simulink model "gm_sampleModel1881_sub"  (R2023a)
settings: Solver=VariableStepAuto  StartTime=0.0  StopTime=10.0  RelTol=1e-3
libraries: simulink x2
settings Model: Creator=user1  LastModifiedBy=user1
settings OptimizationCC: BlockReduction=off  ConditionallyExecuteInputs=off
settings DebuggingCC: InheritedTsInSrcMsg=none

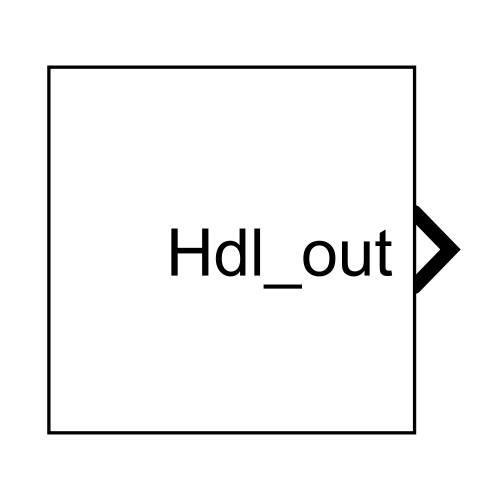
[thumbnail: Simulink's stored preview of the top-level diagram]
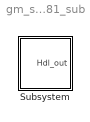
== system gm_sampleModel1881_sub ==
  Subsystem : Subsystem

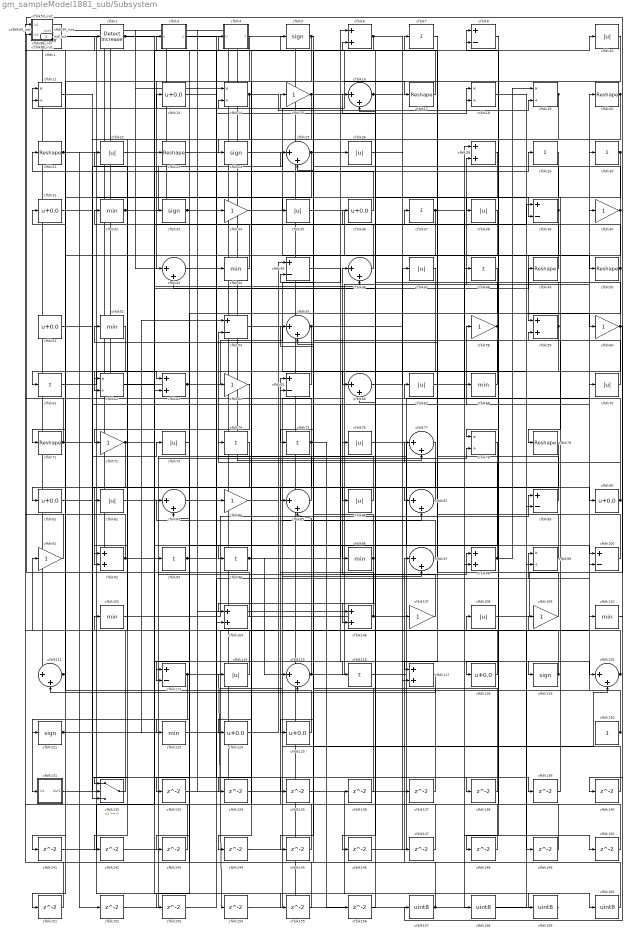
== system gm_sampleModel1881_sub/Subsystem ==
  cfblk1 : simulink/Logic and Bit Operations/Bit Clear  iBit=0
      settings: LibrarySourceBlock=|
      | hdlsllib/Logic and Bit
      | Operations/Bit Clear
  cfblk{10,22,26,35,38,47,67,70,73,76,82,86,108,114} (14 alike) : Abs  OutDataTypeStr=uint8  SaturateOnIntegerOverflow=off
  cfblk{8,39,45,54,65,89,100,113} (8 alike) : Sum  Inputs=+-  OutDataTypeStr=uint8
  cfblk101_inst : Subsystem
  cfblk{32,44,52,68,96,102,110,123} (8 alike) : MinMax  OutDataTypeStr=uint8
  cfblk{6,28,59,63,92,98,104,106,117} (9 alike) : Sum  OutDataTypeStr=uint8
  cfblk105_inst : Subsystem
  cfblk{15,34,40,58,60,64,72,84,91,107,109} (11 alike) : Gain  OutDataTypeStr=uint8
  cfblk{11,14,18..19,62,78,99} (7 alike) : Product  Inputs=*/  OutDataTypeStr=uint8  RndMeth=Zero  SaturateOnIntegerOverflow=on
  cfblk{16,25,43,46,55,66,77,83,85,87,97,111,115,120} (14 alike) : Sum  Inputs=|++  OutDataTypeStr=uint8
  cfblk112_inst : Subsystem
  cfblk{7,29..30,37,48,61,74..75,93..94,116} (11 alike) : Sum  Inputs=+  OutDataTypeStr=uint8
  cfblk{13,31,36,51,81,90,118,124..125} (9 alike) : Bias  Bias=0.0  SaturateOnIntegerOverflow=off
  cfblk{5,24,33,119,121} (5 alike) : Signum
  cfblk130 : Constant  OutDataTypeStr=uint8  SampleTime=-1
  cfblk131 : Subsystem
  cfblk132 : Switch  OutDataTypeStr=uint8  SaturateOnIntegerOverflow=off  InputSameDT=off
  cfblk{133..156} (24 alike) : Delay  SampleTime=1
  cfblk{157..160} (4 alike) : DataTypeConversion  OutDataTypeStr=uint8  SaturateOnIntegerOverflow=off  RndMeth=Floor
  cfblk{17,20..21,23,49..50,71,79} (8 alike) : Reshape
  cfblk2 : simulink/Logic and Bit Operations/Detect Increase  vinit=0.0  OutDataTypeStr=uint8
      settings: LibrarySourceBlock=|
      | hdlsllib/Logic and Bit
      | Operations/Detect
      | Increase
  cfblk3 : Subsystem  mask(Compare To Zero){relop=<=, OutDataTypeStr=uint8, ZeroCross=on}
      mask prompts: relop "Simulink:masks:Operator_MP"; OutDataTypeStr "Simulink:masks:OutputDataType_MP"; ZeroCross "Simulink:masks:EnableZerocrossingDetection_MP"
      mask help: Simulink:masks:CompareToZero_MD
      mask init:
      | OutDataTypeStr = 'uint8';
      | ZeroCross = 'on';
      | blkName = 'sampleModel1881_sub/Subsystem/cfblk3';
      | relop = '<=';
      | setValue = 'fixdt(0, 8)';
      mask TypeOptions relop: == | ~= | < | <= | >= | >
      mask TypeOptions OutDataTypeStr: Simulink:masks:uint8 | Simulink:masks:boolean
      mask Callback ZeroCross: sl('zeroCrossEnable', gcbh);
      mask Display: disp([relop,' 0'])
  cfblk4 : Subsystem  mask(Detect Rise Positive){vinit=double(0), InputProcessing=Elements as channels (sample based), OutDataTypeStr=uint8}
      mask prompts: vinit "Simulink:masks:InitialCondition_MP"; InputProcessing "Simulink:masks:InputProcessing_MP"; OutDataTypeStr "Simulink:masks:OutputDataType_MP"
      mask help: Simulink:masks:DetectRisePositive_MD
      mask init:
      | InputProcessing = 'Elements as channels (sample based)';
      | OutDataTypeStr = 'uint8';
      | vinit = double(0);
      mask TypeOptions InputProcessing: Simulink:masks:ColumnsAsChannelsFrameBased | Simulink:masks:ElementsAsChannelsSampleBased
      mask TypeOptions OutDataTypeStr: Simulink:masks:uint8 | Simulink:masks:boolean
      mask Display: fprintf('U > 0\n&  NOT\nU/z > 0')
  cfblk42_inst : Subsystem
  cfblk53_inst : Subsystem
  cfblk57_inst : Subsystem
  cfblk69_inst : Subsystem
  cfblk80_inst : Subsystem
  cfblk88_inst : Subsystem
  cfblk95_inst : Subsystem
  Hdl_out : Outport  OutDataTypeStr=uint8  SampleTime=1
  wires:
  cfblk1/1 -> cfblk160/1
  cfblk10/1 -> cfblk43/1
  cfblk100/1 -> cfblk52/1
  cfblk101_inst/1(out1) -> cfblk51/1, cfblk23/1
  cfblk102/1 -> cfblk89/1
  cfblk104/1 -> cfblk53_inst/2(in2)
  cfblk105_inst/1(out1) -> cfblk44/1
  cfblk106/1 -> cfblk65/1, cfblk104/1
  cfblk107/1 -> cfblk46/1
  cfblk108/1 -> cfblk80_inst/1(in1)
  cfblk109/1 -> cfblk67/1
  cfblk11/1 -> cfblk132/2
  cfblk110/1 -> cfblk157/1
  cfblk111/1 -> cfblk31/1, cfblk11/1
  cfblk112_inst/1(out1) -> cfblk111/1
  cfblk113/1 -> cfblk154/1, cfblk131/1(In1)
  cfblk114/1 -> cfblk32/1
  cfblk115/1 -> cfblk85/2, cfblk20/1
  cfblk116/1 -> cfblk30/1
  cfblk117/1 -> cfblk111/2
  cfblk118/1 -> cfblk3/1(u)
  cfblk119/1 -> cfblk112_inst/2(in2), cfblk102/1
  cfblk120/1 -> cfblk6/2, cfblk108/1
  cfblk121/1 -> cfblk76/1, cfblk54/1
  cfblk123/1 -> cfblk109/1
  cfblk124/1 -> cfblk45/1
  cfblk125/1 -> cfblk88_inst/2(in2)
  cfblk13/1 -> cfblk114/1
  cfblk130/1 -> cfblk40/1, cfblk15/1
  cfblk131/1(Out1) -> cfblk73/1
  cfblk132/1 -> cfblk91/1
  cfblk133/1 -> cfblk28/2
  cfblk134/1 -> cfblk120/2
  cfblk135/1 -> cfblk159/1
  cfblk136/1 -> cfblk45/2
  cfblk137/1 -> cfblk11/2
  cfblk138/1 -> cfblk55/2
  cfblk139/1 -> cfblk59/2
  cfblk14/1 -> cfblk72/1, cfblk19/2
  cfblk140/1 -> cfblk25/2
  cfblk141/1 -> cfblk63/2
  cfblk142/1 -> cfblk98/1
  cfblk143/1 -> cfblk57_inst/1(in1)
  cfblk144/1 -> cfblk97/2
  cfblk145/1 -> cfblk65/2
  cfblk146/1 -> cfblk99/1
  cfblk147/1 -> cfblk16/2
  cfblk148/1 -> cfblk80_inst/2(in2)
  cfblk149/1 -> cfblk14/2
  cfblk15/1 -> cfblk17/1, cfblk132/3
  cfblk150/1 -> cfblk8/1
  cfblk151/1 -> cfblk95_inst/1(in1)
  cfblk152/1 -> cfblk78/2
  cfblk153/1 -> cfblk100/2
  cfblk154/1 -> cfblk87/2
  cfblk155/1 -> cfblk83/2
  cfblk156/1 -> cfblk66/2
  cfblk157/1 -> cfblk42_inst/1(in1), cfblk115/2
  cfblk158/1 -> cfblk110/1
  cfblk159/1 -> cfblk1/1
  cfblk16/1 -> cfblk119/1, cfblk146/1
  cfblk160/1 -> cfblk97/1
  cfblk17/1 -> cfblk53_inst/1(in1)
  cfblk18/1 -> cfblk60/1
  cfblk19/1 -> cfblk24/1, cfblk118/1
  cfblk2/1 -> cfblk100/1, cfblk155/1
  cfblk20/1 -> cfblk89/2, cfblk148/1
  cfblk21/1 -> cfblk39/2, cfblk152/1
  cfblk22/1 -> cfblk46/2
  cfblk23/1 -> cfblk85/1
  cfblk24/1 -> cfblk50/1
  cfblk25/1 -> cfblk81/1, cfblk124/1
  cfblk26/1 -> cfblk147/1
  cfblk28/1 -> cfblk66/1
  cfblk29/1 -> cfblk86/1
  cfblk3/1(y) -> cfblk34/1
  cfblk30/1 -> cfblk79/1, cfblk106/2
  cfblk31/1 -> cfblk135/1
  cfblk32/1 -> cfblk8/2, cfblk33/1, cfblk7/1
  cfblk33/1 -> cfblk104/2, cfblk139/1
  cfblk34/1 -> cfblk38/1
  cfblk35/1 -> cfblk59/1
  cfblk36/1 -> cfblk21/1
  cfblk37/1 -> cfblk150/1, cfblk94/1
  cfblk38/1 -> cfblk121/1
  cfblk39/1 -> cfblk5/1, cfblk99/2
  cfblk4/1(Y) -> cfblk141/1
  cfblk40/1 -> cfblk132/1, cfblk101_inst/2(in2)
  cfblk42_inst/1(out1) -> cfblk137/1, cfblk136/1
  cfblk43/1 -> cfblk18/1
  cfblk44/1 -> cfblk22/1
  cfblk45/1 -> cfblk120/1
  cfblk46/1 -> cfblk6/1
  cfblk47/1 -> cfblk75/1
  cfblk48/1 -> cfblk143/1
  cfblk49/1 -> cfblk4/1(U)
  cfblk5/1 -> cfblk145/1, cfblk144/1
  cfblk50/1 -> cfblk36/1, cfblk113/2
  cfblk51/1 -> cfblk90/1
  cfblk52/1 -> cfblk61/1
  cfblk53_inst/1(out1) -> cfblk107/1
  cfblk54/1 -> cfblk149/1
  cfblk55/1 -> cfblk92/2, cfblk71/1, cfblk117/2
  cfblk57_inst/1(out1) -> cfblk69_inst/1(in1)
  cfblk58/1 -> cfblk125/1, cfblk2/1
  cfblk59/1 -> cfblk28/1, cfblk62/2
  cfblk6/1 -> cfblk42_inst/2(in2), cfblk138/1
  cfblk60/1 -> cfblk98/2, cfblk105_inst/2(in2), cfblk140/1
  cfblk61/1 -> cfblk63/1
  cfblk62/1 -> cfblk39/1
  cfblk63/1 -> cfblk18/2, Hdl_out/1
  cfblk64/1 -> cfblk142/1
  cfblk65/1 -> cfblk62/1
  cfblk66/1 -> cfblk47/1
  cfblk67/1 -> cfblk58/1
  cfblk68/1 -> cfblk101_inst/1(in1)
  cfblk69_inst/1(out1) -> cfblk77/2, cfblk112_inst/1(in1), cfblk93/1
  cfblk7/1 -> cfblk117/1
  cfblk70/1 -> cfblk16/1
  cfblk71/1 -> cfblk69_inst/2(in2), cfblk25/1
  cfblk72/1 -> cfblk151/1, cfblk116/1
  cfblk73/1 -> cfblk153/1
  cfblk74/1 -> cfblk113/1
  cfblk75/1 -> cfblk57_inst/2(in2), cfblk156/1, cfblk133/1
  cfblk76/1 -> cfblk158/1
  cfblk77/1 -> cfblk92/1
  cfblk78/1 -> cfblk123/1
  cfblk79/1 -> cfblk82/1
  cfblk8/1 -> cfblk78/1
  cfblk80_inst/1(out1) -> cfblk35/1
  cfblk81/1 -> cfblk68/1
  cfblk82/1 -> cfblk48/1
  cfblk83/1 -> cfblk84/1
  cfblk84/1 -> cfblk87/1
  cfblk85/1 -> cfblk54/2
  cfblk86/1 -> cfblk64/1
  cfblk87/1 -> cfblk55/1
  cfblk88_inst/1(out1) -> cfblk26/1
  cfblk89/1 -> cfblk88_inst/1(in1)
  cfblk90/1 -> cfblk43/2, cfblk74/1
  cfblk91/1 -> cfblk105_inst/1(in1)
  cfblk92/1 -> cfblk95_inst/2(in2), cfblk49/1, cfblk29/1
  cfblk93/1 -> cfblk10/1, cfblk96/1
  cfblk94/1 -> cfblk70/1, cfblk115/1
  cfblk95_inst/1(out1) -> cfblk106/1, cfblk14/1
  cfblk96/1 -> cfblk13/1, cfblk134/1
  cfblk97/1 -> cfblk83/1
  cfblk98/1 -> cfblk77/1, cfblk19/1
  cfblk99/1 -> cfblk37/1

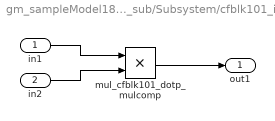
== system gm_sampleModel1881_sub/Subsystem/cfblk101_inst ==
  in1 : Inport  OutDataTypeStr=uint8  SampleTime=1
  in2 : Inport  Port=2  OutDataTypeStr=uint8  SampleTime=1
  mul_cfblk101_dotp_mulcomp : Product  Inputs=**  OutDataTypeStr=uint8  SampleTime=1
  out1 : Outport  OutDataTypeStr=uint8  SampleTime=1
  wires:
  in1/1 -> mul_cfblk101_dotp_mulcomp/1
  in2/1 -> mul_cfblk101_dotp_mulcomp/2
  mul_cfblk101_dotp_mulcomp/1 -> out1/1

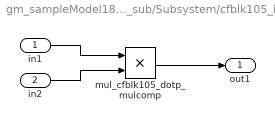
== system gm_sampleModel1881_sub/Subsystem/cfblk105_inst ==
  in1 : Inport  OutDataTypeStr=uint8  SampleTime=1
  in2 : Inport  Port=2  OutDataTypeStr=uint8  SampleTime=1
  mul_cfblk105_dotp_mulcomp : Product  Inputs=**  OutDataTypeStr=uint8  SampleTime=1
  out1 : Outport  OutDataTypeStr=uint8  SampleTime=1
  wires:
  in1/1 -> mul_cfblk105_dotp_mulcomp/1
  in2/1 -> mul_cfblk105_dotp_mulcomp/2
  mul_cfblk105_dotp_mulcomp/1 -> out1/1

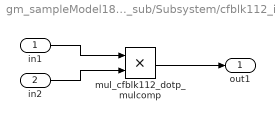
== system gm_sampleModel1881_sub/Subsystem/cfblk112_inst ==
  in1 : Inport  OutDataTypeStr=uint8  SampleTime=1
  in2 : Inport  Port=2  OutDataTypeStr=uint8  SampleTime=1
  mul_cfblk112_dotp_mulcomp : Product  Inputs=**  OutDataTypeStr=uint8  SampleTime=1
  out1 : Outport  OutDataTypeStr=uint8  SampleTime=1
  wires:
  in1/1 -> mul_cfblk112_dotp_mulcomp/1
  in2/1 -> mul_cfblk112_dotp_mulcomp/2
  mul_cfblk112_dotp_mulcomp/1 -> out1/1

== system gm_sampleModel1881_sub/Subsystem/cfblk131 ==
  In1 : Inport  OutDataTypeStr=uint8  PortDimensions=1  SampleTime=1
  Out1 : Outport  SampleTime=1
  wires:
  In1/1 -> Out1/1

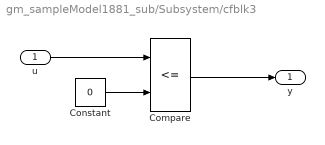
== system gm_sampleModel1881_sub/Subsystem/cfblk3 ==
  u : Inport  OutDataTypeStr=uint8  SampleTime=1
  Compare : RelationalOperator  Operator=<=  OutDataTypeStr=fixdt(0, 8)
  Constant : Constant  DisableCoverage=on  Value=0  OutDataTypeStr=Inherit: Inherit via back propagation  SampleTime=-1  PreserveConstantTs=on
  y : Outport  SampleTime=1
  wires:
  u/1 -> Compare/1
  Compare/1 -> y/1
  Constant/1 -> Compare/2

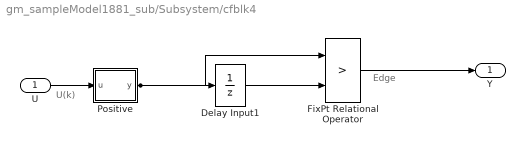
== system gm_sampleModel1881_sub/Subsystem/cfblk4 ==
  note: U(k)
  note: Edge
  U : Inport  OutDataTypeStr=uint8  SampleTime=1
  Delay Input1 : UnitDelay  Description=Store in Global RAM  DisableCoverage=on  InitialCondition=vinit  SampleTime=-1  HasFrameUpgradeWarning=on
  FixPt Relational Operator : RelationalOperator  Operator=>  OutDataTypeStr=fixdt(0, 8)  ZeroCross=off  InputSameDT=off
  Positive : Subsystem  mask(Compare To Zero){relop=>, OutDataTypeStr=boolean, ZeroCross=off}
      mask prompts: relop "Simulink:masks:Operator_MP"; OutDataTypeStr "Simulink:masks:OutputDataType_MP"; ZeroCross "Simulink:masks:EnableZerocrossingDetection_MP"
      mask help: Simulink:masks:CompareToZero_MD
      mask init:
      | OutDataTypeStr = 'boolean';
      | ZeroCross = 'off';
      | blkName = 'sampleModel1881_sub/Subsystem/cfblk4/Positive';
      | relop = '>';
      | setValue = 'boolean';
      mask TypeOptions relop: == | ~= | < | <= | >= | >
      mask TypeOptions OutDataTypeStr: Simulink:masks:uint8 | Simulink:masks:boolean
      mask Callback ZeroCross: sl('zeroCrossEnable', gcbh);
      mask Display: disp([relop,' 0'])
  Y : Outport  SampleTime=1
  wires:
  U/1 -> Positive/1(u)
  Delay Input1/1 -> FixPt Relational Operator/2
  FixPt Relational Operator/1 -> Y/1
  Positive/1(y) -> FixPt Relational Operator/1, Delay Input1/1

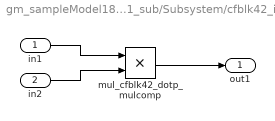
== system gm_sampleModel1881_sub/Subsystem/cfblk42_inst ==
  in1 : Inport  OutDataTypeStr=uint8  SampleTime=1
  in2 : Inport  Port=2  OutDataTypeStr=uint8  SampleTime=1
  mul_cfblk42_dotp_mulcomp : Product  Inputs=**  OutDataTypeStr=uint8  SampleTime=1
  out1 : Outport  OutDataTypeStr=uint8  SampleTime=1
  wires:
  in1/1 -> mul_cfblk42_dotp_mulcomp/1
  in2/1 -> mul_cfblk42_dotp_mulcomp/2
  mul_cfblk42_dotp_mulcomp/1 -> out1/1

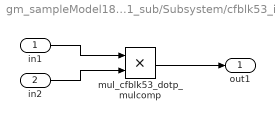
== system gm_sampleModel1881_sub/Subsystem/cfblk53_inst ==
  in1 : Inport  OutDataTypeStr=uint8  SampleTime=1
  in2 : Inport  Port=2  OutDataTypeStr=uint8  SampleTime=1
  mul_cfblk53_dotp_mulcomp : Product  Inputs=**  OutDataTypeStr=uint8  SampleTime=1
  out1 : Outport  OutDataTypeStr=uint8  SampleTime=1
  wires:
  in1/1 -> mul_cfblk53_dotp_mulcomp/1
  in2/1 -> mul_cfblk53_dotp_mulcomp/2
  mul_cfblk53_dotp_mulcomp/1 -> out1/1

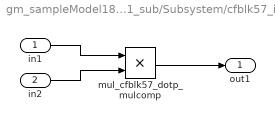
== system gm_sampleModel1881_sub/Subsystem/cfblk57_inst ==
  in1 : Inport  OutDataTypeStr=uint8  SampleTime=1
  in2 : Inport  Port=2  OutDataTypeStr=uint8  SampleTime=1
  mul_cfblk57_dotp_mulcomp : Product  Inputs=**  OutDataTypeStr=uint8  SampleTime=1
  out1 : Outport  OutDataTypeStr=uint8  SampleTime=1
  wires:
  in1/1 -> mul_cfblk57_dotp_mulcomp/1
  in2/1 -> mul_cfblk57_dotp_mulcomp/2
  mul_cfblk57_dotp_mulcomp/1 -> out1/1

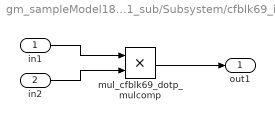
== system gm_sampleModel1881_sub/Subsystem/cfblk69_inst ==
  in1 : Inport  OutDataTypeStr=uint8  SampleTime=1
  in2 : Inport  Port=2  OutDataTypeStr=uint8  SampleTime=1
  mul_cfblk69_dotp_mulcomp : Product  Inputs=**  OutDataTypeStr=uint8  SampleTime=1
  out1 : Outport  OutDataTypeStr=uint8  SampleTime=1
  wires:
  in1/1 -> mul_cfblk69_dotp_mulcomp/1
  in2/1 -> mul_cfblk69_dotp_mulcomp/2
  mul_cfblk69_dotp_mulcomp/1 -> out1/1

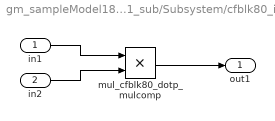
== system gm_sampleModel1881_sub/Subsystem/cfblk80_inst ==
  in1 : Inport  OutDataTypeStr=uint8  SampleTime=1
  in2 : Inport  Port=2  OutDataTypeStr=uint8  SampleTime=1
  mul_cfblk80_dotp_mulcomp : Product  Inputs=**  OutDataTypeStr=uint8  SampleTime=1
  out1 : Outport  OutDataTypeStr=uint8  SampleTime=1
  wires:
  in1/1 -> mul_cfblk80_dotp_mulcomp/1
  in2/1 -> mul_cfblk80_dotp_mulcomp/2
  mul_cfblk80_dotp_mulcomp/1 -> out1/1

== system gm_sampleModel1881_sub/Subsystem/cfblk88_inst ==
  in1 : Inport  OutDataTypeStr=uint8  SampleTime=1
  in2 : Inport  Port=2  OutDataTypeStr=uint8  SampleTime=1
  mul_cfblk88_dotp_mulcomp : Product  Inputs=**  OutDataTypeStr=uint8  SampleTime=1
  out1 : Outport  OutDataTypeStr=uint8  SampleTime=1
  wires:
  in1/1 -> mul_cfblk88_dotp_mulcomp/1
  in2/1 -> mul_cfblk88_dotp_mulcomp/2
  mul_cfblk88_dotp_mulcomp/1 -> out1/1

== system gm_sampleModel1881_sub/Subsystem/cfblk95_inst ==
  in1 : Inport  OutDataTypeStr=uint8  SampleTime=1
  in2 : Inport  Port=2  OutDataTypeStr=uint8  SampleTime=1
  mul_cfblk95_dotp_mulcomp : Product  Inputs=**  OutDataTypeStr=uint8  SampleTime=1
  out1 : Outport  OutDataTypeStr=uint8  SampleTime=1
  wires:
  in1/1 -> mul_cfblk95_dotp_mulcomp/1
  in2/1 -> mul_cfblk95_dotp_mulcomp/2
  mul_cfblk95_dotp_mulcomp/1 -> out1/1

== system gm_sampleModel1881_sub/Subsystem/cfblk4/Positive ==
  u : Inport  OutDataTypeStr=uint8  SampleTime=1
  Compare : RelationalOperator  Operator=>  OutDataTypeStr=boolean  ZeroCross=off
  Constant : Constant  DisableCoverage=on  Value=0  OutDataTypeStr=Inherit: Inherit via back propagation  SampleTime=-1  PreserveConstantTs=on
  y : Outport  SampleTime=1
  wires:
  u/1 -> Compare/1
  Compare/1 -> y/1
  Constant/1 -> Compare/2
